simulink model "gm_sampleModel1420_3_sub_sub"  (R2023a)
settings: Solver=VariableStepAuto  StartTime=0.0  StopTime=10.0  RelTol=1e-3
libraries: hdlsllib x5, simulink x2
settings Model: Creator=user1  LastModifiedBy=user1
settings OptimizationCC: BlockReduction=off  ConditionallyExecuteInputs=off
settings DebuggingCC: InheritedTsInSrcMsg=none

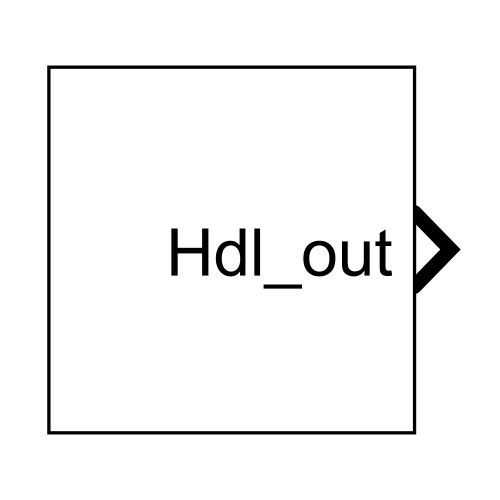
[thumbnail: Simulink's stored preview of the top-level diagram]
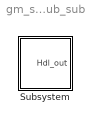
== system gm_sampleModel1420_3_sub_sub ==
  Subsystem : Subsystem

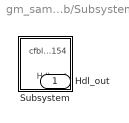
== system gm_sampleModel1420_3_sub_sub/Subsystem ==
  Subsystem : Subsystem
  Hdl_out : Outport  OutDataTypeStr=uint8

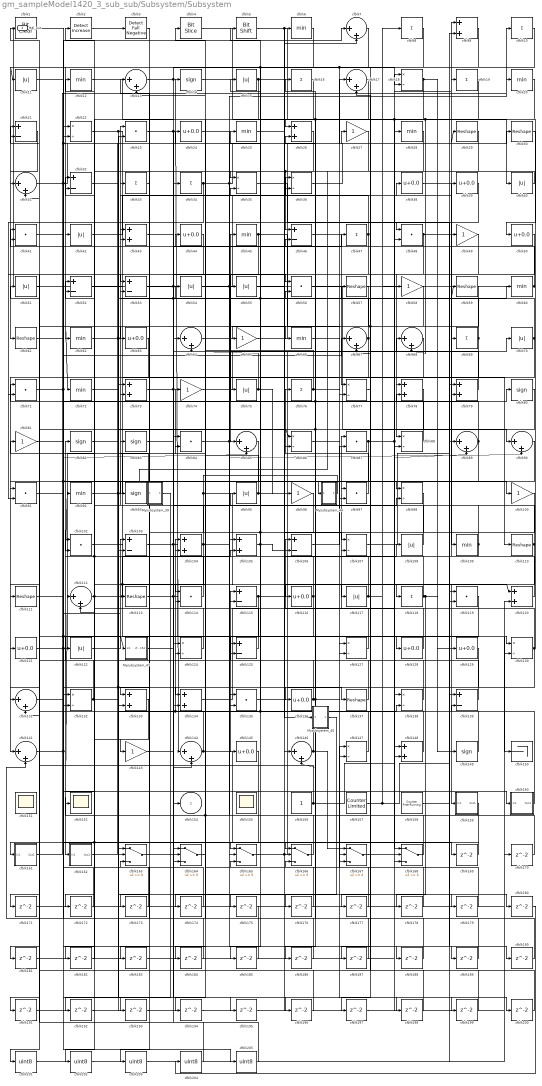
== system gm_sampleModel1420_3_sub_sub/Subsystem/Subsystem ==
  Mysubsystem_39 : Subsystem  TreatAsAtomicUnit=on  RTWFcnName=Mysubsystem_39
      settings: RTWFcnNameOpts=User specified  RTWFileNameOpts=Use function name
  Mysubsystem_40 : Subsystem  TreatAsAtomicUnit=on  RTWFcnName=Mysubsystem_40
      settings: RTWFcnNameOpts=User specified  RTWFileNameOpts=Use function name
  Mysubsystem_44 : Subsystem  TreatAsAtomicUnit=on  RTWFcnName=Mysubsystem_44
      settings: RTWFcnNameOpts=User specified  RTWFileNameOpts=Use function name
  Mysubsystem_47 : Subsystem  TreatAsAtomicUnit=on  RTWFcnName=Mysubsystem_47
      settings: RTWFcnNameOpts=User specified  RTWFileNameOpts=Use function name
  cfblk1 : simulink/Logic and Bit Operations/Bit Clear  iBit=0
      settings: LibrarySourceBlock=|
      | hdlsllib/Logic and Bit
      | Operations/Bit Clear
  cfblk{8,10,16,19,33..34,47,69,76,118} (10 alike) : Sum  Inputs=+  OutDataTypeStr=uint8
  cfblk{27,49,58,65,74,81,96,100,143} (9 alike) : Gain  OutDataTypeStr=uint8
  cfblk{23,41,48,56,71,84,87,91,97,102,114,119,135} (13 alike) : DotProduct  OutDataTypeStr=uint8
  cfblk{21,32,46,52..53,103,106,115,125,139} (10 alike) : Sum  Inputs=+-  OutDataTypeStr=uint8
  cfblk{9,26,43,73,78..79,104..105,120,133..134,148} (12 alike) : Sum  OutDataTypeStr=uint8
  cfblk{18,22,35..36,77,86,88,98,107,124,127,130,132,138,147} (15 alike) : Product  Inputs=*/  OutDataTypeStr=uint8  RndMeth=Zero  SaturateOnIntegerOverflow=on
  cfblk{11,15,40,42,51,54..55,70,75,95,108,117,122} (13 alike) : Abs  OutDataTypeStr=uint8  SaturateOnIntegerOverflow=off
  cfblk{6,12,20,25,28,45,60,62,66,72,92,109} (12 alike) : MinMax  OutDataTypeStr=uint8
  cfblk{29..30,57,59,61,110..111,113,137} (9 alike) : Reshape
  cfblk{7,13,17,31,64,67..68,85,89..90,112,131,141,144,146} (15 alike) : Sum  Inputs=|++  OutDataTypeStr=uint8
  cfblk{24,38..39,44,50,63,116,121,128..129,136,145} (12 alike) : Bias  Bias=0.0  SaturateOnIntegerOverflow=off
  cfblk{14,80,82..83,93,149} (6 alike) : Signum
  cfblk150 : Terminator
  cfblk151 : Scope
      settings: Floating=on
  cfblk152 : Scope
  cfblk155 : Scope
      settings: Floating=on
  cfblk156 : Constant  OutDataTypeStr=uint8  SampleTime=-1
  cfblk157 : hdlsllib/Sources/Counter Limited  uplimit=7  tsamp=-1
  cfblk158 : hdlsllib/Sources/Counter Free-Running  NumBits=16  tsamp=-1
  cfblk159 : Subsystem
      settings: LibrarySourceBlock=|
      | hdlsllib/Ports &
      | Subsystems/Subsystem
  cfblk160 : Subsystem
      settings: LibrarySourceBlock=|
      | hdlsllib/Ports &
      | Subsystems/Subsystem
  cfblk161 : Subsystem
      settings: LibrarySourceBlock=|
      | hdlsllib/Ports &
      | Subsystems/Subsystem
  cfblk162 : Subsystem
      settings: LibrarySourceBlock=|
      | hdlsllib/Ports &
      | Subsystems/Subsystem
  cfblk{163..168} (6 alike) : Switch  OutDataTypeStr=uint8  SaturateOnIntegerOverflow=off  InputSameDT=off
  cfblk{169..200} (32 alike) : Delay  SampleTime=1
  cfblk2 : simulink/Logic and Bit Operations/Detect Increase  vinit=0.0  OutDataTypeStr=uint8
      settings: LibrarySourceBlock=|
      | hdlsllib/Logic and Bit
      | Operations/Detect
      | Increase
  cfblk{201..205} (5 alike) : DataTypeConversion  OutDataTypeStr=uint8  SaturateOnIntegerOverflow=off  RndMeth=Floor
  cfblk3 : hdlsllib/Logic and Bit Operations/Detect Fall Negative  vinit=0  OutDataTypeStr=uint8
  cfblk4 : hdlsllib/Logic and Bit Operations/Bit Slice  lidx=7  ridx=0
  cfblk5 : hdlsllib/Logic and Bit Operations/Bit Shift  mode=Shift Left Logical  N=0
  cfblk154 : Outport  OutDataTypeStr=uint8  VectorParamsAs1DForOutWhenUnconnected=off
  Hdl_out : Outport  Port=2  OutDataTypeStr=uint8
  wires:
  cfblk165/1 -> cfblk108/1, cfblk70/1
  cfblk144/1 -> cfblk41/2, cfblk166/1
  cfblk139/1 -> cfblk115/1
  cfblk6/1 -> cfblk61/1
  cfblk75/1 -> cfblk64/2, cfblk96/1
  cfblk162/1(Out1) -> cfblk27/1
  cfblk59/1 -> cfblk197/1, cfblk72/1
  cfblk54/1 -> cfblk188/1, cfblk38/1
  cfblk138/1 -> cfblk82/1
  cfblk161/1(Out1) -> cfblk10/1
  cfblk62/1 -> cfblk60/1, cfblk130/1
  cfblk10/1 -> cfblk62/1
  cfblk127/1 -> cfblk87/1
  cfblk130/1 -> cfblk67/2, cfblk164/3, cfblk26/1
  cfblk115/1 -> cfblk7/2, cfblk162/1(In1)
  cfblk22/1 -> cfblk86/2, cfblk118/1
  cfblk70/1 -> cfblk53/2, cfblk141/1
  cfblk48/1 -> cfblk190/1, cfblk88/1
  cfblk23/1 -> cfblk167/3, cfblk144/1
  cfblk116/1 -> cfblk191/1, cfblk43/1
  cfblk134/1 -> cfblk28/1
  cfblk63/1 -> cfblk161/1(In1)
  cfblk97/1 -> cfblk76/1
  cfblk93/1 -> cfblk23/1
  cfblk146/1 -> cfblk167/1, cfblk21/1, cfblk25/1
  cfblk56/1 -> cfblk90/1
  cfblk148/1 -> cfblk43/2, cfblk104/1
  cfblk121/1 -> cfblk67/1, cfblk74/1
  cfblk16/1 -> cfblk53/1
  cfblk110/1 -> cfblk136/1, cfblk83/1
  cfblk95/1 -> cfblk98/1, cfblk44/1
  cfblk4/1 -> cfblk127/1
  cfblk168/1 -> cfblk114/2, cfblk112/1
  cfblk87/1 -> cfblk175/1, cfblk19/1, cfblk89/2
  cfblk5/1 -> cfblk107/1, cfblk168/1
  cfblk117/1 -> cfblk58/1, cfblk2/1, cfblk92/1
  cfblk26/1 -> cfblk165/1
  cfblk109/1 -> cfblk107/2, cfblk97/1
  cfblk85/1 -> cfblk121/1
  cfblk46/1 -> cfblk77/1
  cfblk120/1 -> cfblk9/1
  cfblk104/1 -> cfblk20/1, cfblk122/1, cfblk73/2
  cfblk50/1 -> cfblk85/1
  cfblk88/1 -> cfblk45/1
  cfblk57/1 -> cfblk91/1
  cfblk12/1 -> cfblk64/1
  cfblk51/1 -> cfblk131/1
  cfblk125/1 -> cfblk71/1
  cfblk106/1 -> cfblk87/2
  cfblk65/1 -> cfblk17/1
  cfblk2/1 -> cfblk3/1
  cfblk67/1 -> cfblk15/1, cfblk115/2
  cfblk112/1 -> cfblk12/1, cfblk34/1, cfblk147/2
  cfblk122/1 -> cfblk103/1
  cfblk34/1 -> cfblk71/2, cfblk18/1, cfblk55/1
  cfblk11/1 -> cfblk164/2
  cfblk38/1 -> cfblk109/1
  cfblk149/1 -> cfblk54/1
  cfblk64/1 -> cfblk66/1
  cfblk39/1 -> cfblk134/1
  cfblk17/1 -> cfblk173/1, cfblk146/2
  cfblk47/1 -> cfblk13/1, cfblk91/2
  cfblk163/1 -> cfblk105/2
  cfblk156/1 -> cfblk48/2, cfblk131/2
  cfblk90/1 -> cfblk132/2
  cfblk31/1 -> cfblk7/1, cfblk14/1
  cfblk158/1 -> cfblk139/1
  cfblk45/1 -> cfblk103/2, cfblk97/2
  cfblk159/1(Out1) -> cfblk182/1, cfblk181/1
  cfblk27/1 -> cfblk184/1, cfblk46/1
  cfblk108/1 -> cfblk52/1
  cfblk83/1 -> cfblk59/1, cfblk36/1
  cfblk103/1 -> cfblk57/1, cfblk150/1
  cfblk86/1 -> cfblk100/1
  cfblk113/1 -> cfblk98/2, cfblk128/1
  cfblk84/1 -> cfblk79/2, cfblk90/2
  cfblk124/1 -> cfblk81/1
  cfblk166/1 -> cfblk33/1
  cfblk15/1 -> cfblk193/1, cfblk40/1
  cfblk135/1 -> cfblk137/1
  cfblk36/1 -> cfblk30/1
  cfblk72/1 -> cfblk196/1, cfblk134/2
  cfblk92/1 -> cfblk167/2, cfblk24/1
  cfblk132/1 -> cfblk138/2, cfblk51/1
  cfblk29/1 -> cfblk48/1
  cfblk76/1 -> cfblk179/1, cfblk13/2
  cfblk79/1 -> cfblk65/1
  cfblk105/1 -> cfblk106/2, cfblk5/1
  cfblk61/1 -> cfblk160/1(In1), Mysubsystem_47/1(In1), Mysubsystem_44/1(In1)
  cfblk102/1 -> cfblk120/1, cfblk145/1
  cfblk98/1 -> cfblk125/2, cfblk135/1
  cfblk69/1 -> cfblk194/1, cfblk35/2, cfblk4/1
  cfblk21/1 -> cfblk31/1
  cfblk43/1 -> cfblk39/1
  cfblk73/1 -> cfblk195/1, cfblk69/1
  cfblk58/1 -> cfblk78/1
  cfblk167/1 -> cfblk138/1
  cfblk141/1 -> cfblk113/1, cfblk163/2
  cfblk74/1 -> cfblk68/1
  cfblk52/1 -> cfblk110/1
  cfblk81/1 -> cfblk80/1
  cfblk71/1 -> cfblk85/2, cfblk29/1, cfblk22/2
  cfblk82/1 -> cfblk75/1
  cfblk164/1 -> cfblk84/2
  cfblk33/1 -> cfblk63/1
  cfblk107/1 -> cfblk49/1
  cfblk30/1 -> cfblk50/1
  cfblk53/1 -> cfblk199/1, cfblk56/1
  cfblk131/1 -> cfblk78/2
  cfblk96/1 -> cfblk133/1
  cfblk80/1 -> cfblk93/1
  cfblk128/1 -> cfblk106/1
  cfblk13/1 -> cfblk180/1, cfblk18/2
  cfblk114/1 -> cfblk52/2
  cfblk19/1 -> cfblk68/2, cfblk125/1
  cfblk143/1 -> cfblk47/1
  cfblk89/1 -> cfblk135/2, cfblk56/2, cfblk32/1
  cfblk20/1 -> cfblk114/1, cfblk88/2
  cfblk9/1 -> cfblk127/2, cfblk35/1, cfblk11/1
  cfblk147/1 -> cfblk102/1
  cfblk24/1 -> cfblk77/2
  cfblk18/1 -> cfblk129/1, cfblk42/1
  cfblk68/1 -> cfblk116/1, cfblk86/1
  cfblk44/1 -> cfblk111/1
  cfblk35/1 -> cfblk89/1
  cfblk42/1 -> cfblk6/1
  cfblk100/1 -> cfblk143/1
  cfblk41/1 -> cfblk133/2
  cfblk136/1 -> cfblk95/1, cfblk200/1, cfblk16/1
  cfblk160/1(Out1) -> cfblk139/2
  cfblk60/1 -> Hdl_out/1, cfblk41/1
  cfblk28/1 -> cfblk152/1
  cfblk14/1 -> cfblk148/1
  cfblk55/1 -> cfblk36/2
  cfblk118/1 -> cfblk32/2, cfblk178/1, cfblk149/1
  cfblk157/1 -> cfblk8/1, cfblk9/2
  cfblk8/1 -> cfblk117/1
  cfblk137/1 -> cfblk46/2
  cfblk66/1 -> cfblk169/1
  cfblk169/1 -> cfblk165/2
  cfblk170/1 -> cfblk105/1
  cfblk78/1 -> cfblk171/1
  cfblk171/1 -> cfblk130/2
  cfblk133/1 -> cfblk172/1
  cfblk172/1 -> cfblk132/1
  cfblk173/1 -> cfblk163/1
  cfblk174/1 -> cfblk112/2
  cfblk175/1 -> cfblk141/2
  cfblk32/1 -> cfblk176/1
  cfblk176/1 -> cfblk124/2
  cfblk77/1 -> cfblk177/1
  cfblk177/1 -> cfblk166/3
  cfblk178/1 -> cfblk147/1
  cfblk179/1 -> cfblk165/3
  cfblk181/1 -> cfblk144/2
  cfblk182/1 -> cfblk102/2
  cfblk183/1 -> cfblk148/2
  cfblk184/1 -> cfblk163/3
  cfblk7/1 -> cfblk185/1
  cfblk185/1 -> cfblk22/1
  cfblk129/1 -> cfblk186/1
  cfblk186/1 -> cfblk84/1
  cfblk49/1 -> cfblk187/1
  cfblk187/1 -> cfblk26/2
  cfblk188/1 -> cfblk104/2
  cfblk91/1 -> cfblk189/1
  cfblk189/1 -> cfblk73/1
  cfblk190/1 -> cfblk21/2
  cfblk191/1 -> cfblk164/1
  cfblk192/1 -> cfblk23/2
  cfblk193/1 -> cfblk120/2
  cfblk194/1 -> cfblk79/1
  cfblk195/1 -> cfblk146/1
  cfblk196/1 -> cfblk166/2
  cfblk197/1 -> cfblk168/3
  cfblk111/1 -> cfblk198/1
  cfblk198/1 -> cfblk168/2
  cfblk199/1 -> cfblk17/2
  cfblk200/1 -> cfblk31/2
  cfblk119/1 -> cfblk201/1
  cfblk201/1 -> cfblk170/1
  cfblk145/1 -> cfblk202/1
  cfblk202/1 -> cfblk119/1
  cfblk3/1 -> cfblk203/1
  cfblk203/1 -> cfblk119/2
  cfblk180/1 -> cfblk204/1
  cfblk204/1 -> cfblk1/1
  cfblk1/1 -> cfblk205/1
  cfblk205/1 -> cfblk124/1
  cfblk40/1 -> Mysubsystem_39/1(In1)
  Mysubsystem_39/1(Out1) -> cfblk192/1
  cfblk25/1 -> Mysubsystem_40/1(In1)
  Mysubsystem_40/1(Out1) -> cfblk174/1
  Mysubsystem_44/1(Out1) -> cfblk183/1, cfblk159/1(In1)
  Mysubsystem_47/1(cfblk154) -> cfblk154/1

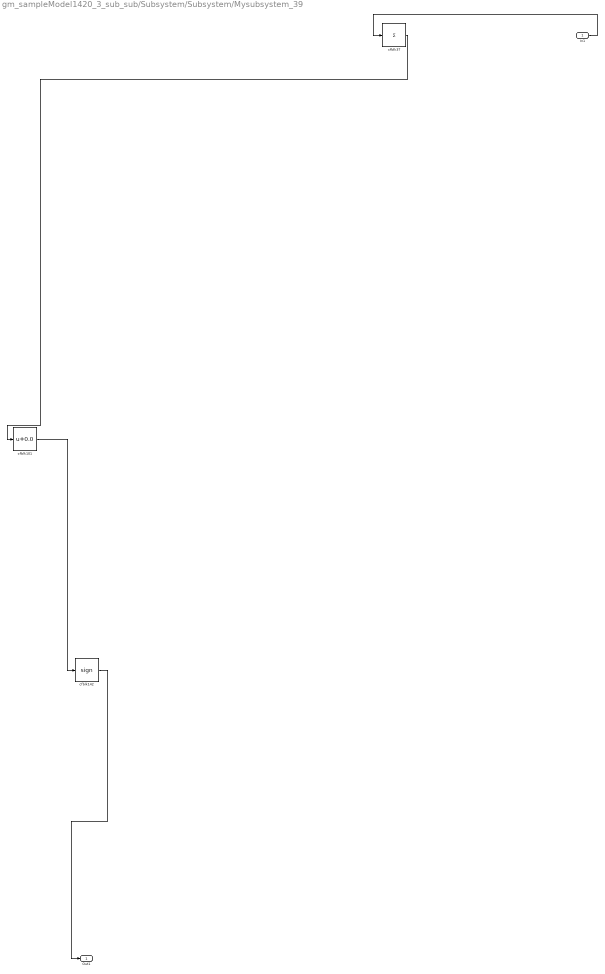
== system gm_sampleModel1420_3_sub_sub/Subsystem/Subsystem/Mysubsystem_39 ==
  In1 : Inport
  cfblk101 : Bias  Bias=0.0  SaturateOnIntegerOverflow=off
  cfblk142 : Signum
  cfblk37 : Sum  Inputs=+
  Out1 : Outport
  wires:
  In1/1 -> cfblk37/1
  cfblk142/1 -> Out1/1
  cfblk37/1 -> cfblk101/1
  cfblk101/1 -> cfblk142/1

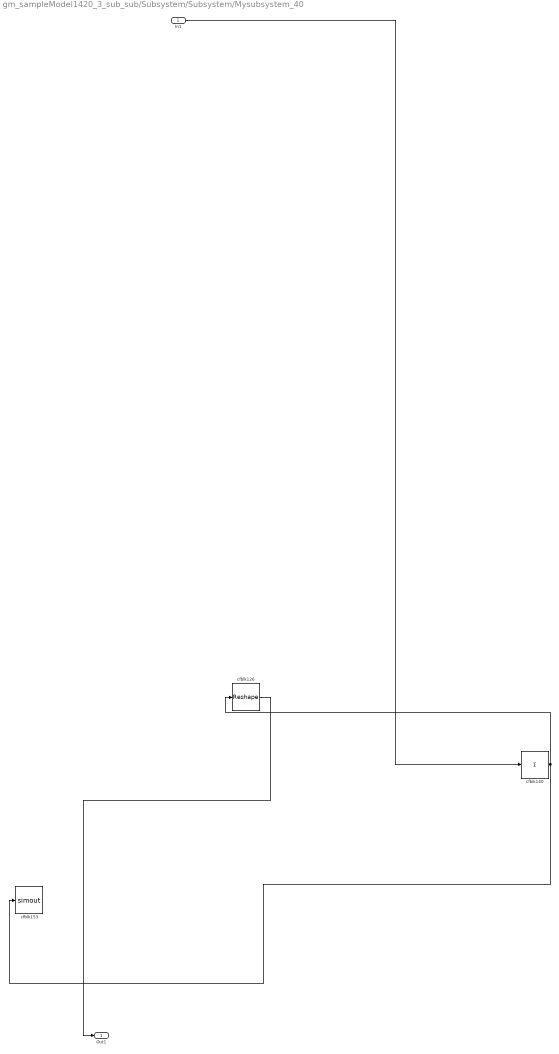
== system gm_sampleModel1420_3_sub_sub/Subsystem/Subsystem/Mysubsystem_40 ==
  In1 : Inport
  cfblk126 : Reshape
  cfblk140 : Sum  Inputs=+
  cfblk153 : ToWorkspace  VariableName=simout  SaveFormat=Timeseries  SampleTime=-1
  Out1 : Outport
  wires:
  cfblk126/1 -> Out1/1
  In1/1 -> cfblk140/1
  cfblk140/1 -> cfblk126/1, cfblk153/1

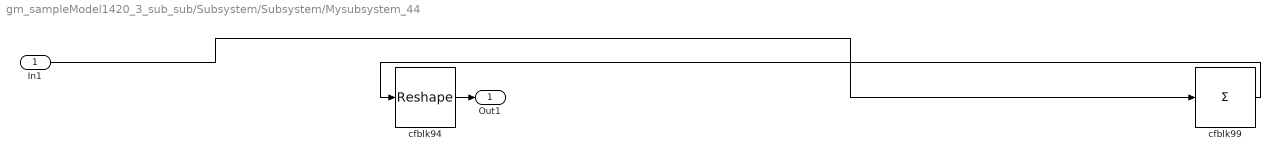
== system gm_sampleModel1420_3_sub_sub/Subsystem/Subsystem/Mysubsystem_44 ==
  In1 : Inport
  cfblk94 : Reshape
  cfblk99 : Sum  Inputs=+
  Out1 : Outport
  wires:
  cfblk94/1 -> Out1/1
  In1/1 -> cfblk99/1
  cfblk99/1 -> cfblk94/1

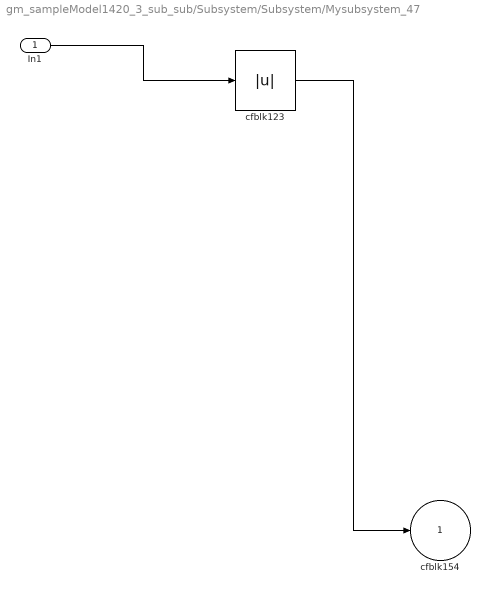
== system gm_sampleModel1420_3_sub_sub/Subsystem/Subsystem/Mysubsystem_47 ==
  In1 : Inport
  cfblk123 : Abs  SaturateOnIntegerOverflow=off
  cfblk154 : Outport  VectorParamsAs1DForOutWhenUnconnected=off
  wires:
  cfblk123/1 -> cfblk154/1
  In1/1 -> cfblk123/1

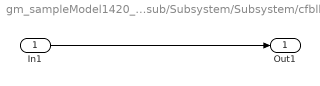
== system gm_sampleModel1420_3_sub_sub/Subsystem/Subsystem/cfblk159 ==
  In1 : Inport
  Out1 : Outport
  wires:
  In1/1 -> Out1/1

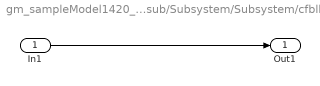
== system gm_sampleModel1420_3_sub_sub/Subsystem/Subsystem/cfblk160 ==
  In1 : Inport
  Out1 : Outport
  wires:
  In1/1 -> Out1/1

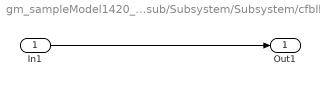
== system gm_sampleModel1420_3_sub_sub/Subsystem/Subsystem/cfblk161 ==
  In1 : Inport
  Out1 : Outport
  wires:
  In1/1 -> Out1/1

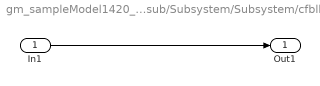
== system gm_sampleModel1420_3_sub_sub/Subsystem/Subsystem/cfblk162 ==
  In1 : Inport
  Out1 : Outport
  wires:
  In1/1 -> Out1/1
